simulink subsystem "ramp_generator"  (R2020a)
settings: Solver=VariableStepAuto  StartTime=0.0  StopTime=10.0  RelTol=1e-3
undefined symbols (not defined in the file): misu_Ts
settings Model: Creator=andrea  LastModifiedBy=stefano

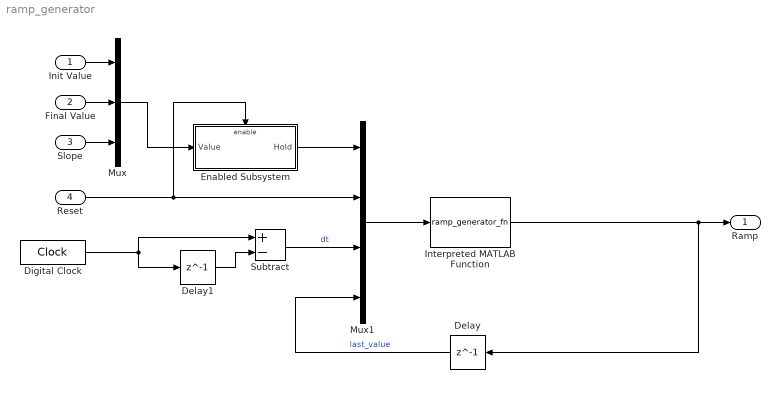
== system ramp_generator ==
  "Init Value " : Inport
  Final Value : Inport  Port=2
  Slope : Inport  Port=3
  Reset : Inport  Port=4
  Delay : Delay  DelayLength=1  SampleTime=misu_Ts
  Delay1 : Delay  DelayLength=1
  Digital Clock : DigitalClock  SampleTime=misu_Ts
  Enabled Subsystem : Subsystem  TreatAsAtomicUnit=on
  Interpreted MATLAB Function : MATLABFcn  MATLABFcn=ramp_generator_fn  OutputDimensions=1
  Mux : Mux  Inputs=3
  Mux1 : Mux
  Subtract : Sum  Inputs=+-
  Ramp : Outport
  wires:
  Reset/1 -> Mux1/2, Enabled Subsystem/Enable
  "Init Value "/1 -> Mux/1
  Delay/1 -> Mux1/4  "last_value"
  Slope/1 -> Mux/3
  Final Value/1 -> Mux/2
  Mux/1 -> Enabled Subsystem/1(Value)
  Enabled Subsystem/1(Hold) -> Mux1/1
  Mux1/1 -> Interpreted MATLAB Function/1
  Digital Clock/1 -> Subtract/1, Delay1/1
  Delay1/1 -> Subtract/2
  Subtract/1 -> Mux1/3  "dt"
  Interpreted MATLAB Function/1 -> Delay/1, Ramp/1

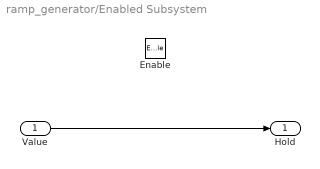
== system ramp_generator/Enabled Subsystem ==
  Value : Inport
  Enable : EnablePort
  Hold : Outport
  wires:
  Value/1 -> Hold/1
